simulink model "Modell_13_1_v2"  (R2018a)
settings: Solver=VariableStepAuto  StartTime=0.0  StopTime=10  MaxStep=0.001  RelTol=1e-3
libraries: simulink x2
settings Model: Creator=Uni  LastModifiedBy=Uni

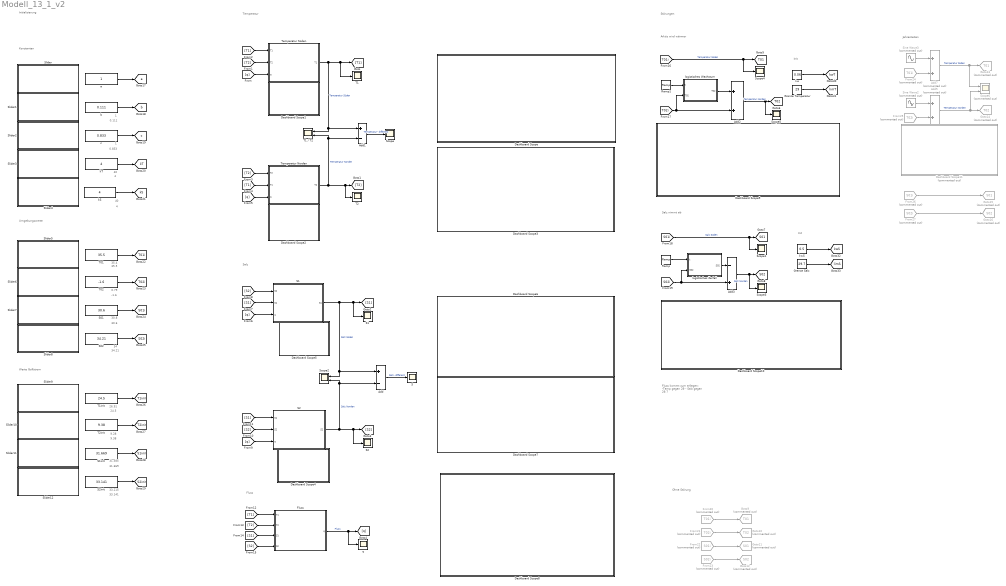
== system Modell_13_1_v2 ==
  note: 35.5
  note: -1.6
  note: 30.6
  note: 34.21
  note: 24.5
  note: 9.38
  note: 31.669
  note: 33.141
  note: 0.111
  note: 0.833
  note: 4
  note: 4
  note: Fluss kommt zum erliegen:
      | -Temp gegen 29
      | - Salz gegen 29.7
  note: Salz nimmt ab
  note: Ohne Störung
  note: Störungen
  note: 9.28
  note: 26.91
  note: 1
  note: 1
  note: 40
  note: 40
  note: 0.79
  note: 35.4
  note: 30.8
  note: 34
  note: 33.215
  note: 31.585
  note: Werte Golfstrom
  note: Umgebungswerte
  note: Konstanten
  note: Initialisierung
  note: Temperatur
  note: Salz
  note: Fluss
  note: Arktis wird wärmer
  note: Jahreszeiten
  note: Init
  note: Init
  Add : Sum  Inputs=+-
  Add1 : Sum  Inputs=+-
  Add2 : Sum
  Add3 : Sum  Inputs=-+
  Add5 : Sum  Commented=on
  Add7 : Sum  Commented=on
  Dashboard Scope : Subsystem  DialogController=hmiCreateDDGDialog  IsWebBlock=on  mask(MWDashboardBlock){webBlockId=232e5835-4ce7-4c9d-ab38-ef92145eaec7, webBlockType=sdiscope, ShowInitialText=on, HMISrcModelName=Modell_13_1_v2}
      mask prompts: webBlockId "WebBlock Id"; webBlockType "WebBlock Type"; HMISrcModelName "Source Model"
      mask help: SimulinkHMI:dialogs:HMIScopeDialogDesc
      mask Help: helpview([docroot '/mapfiles/simulink.map'], 'hmi_scope')
      mask Display:
      | if strcmp(get_param(bdroot(gcb),'BlockDiagramType'), 'library')
      |     image([(matlabroot) '/toolbox/simulink/hmi/icons/DashboardScope.png']);
      | end
  Dashboard Scope1 : Subsystem  DialogController=hmiCreateDDGDialog  IsWebBlock=on  mask(MWDashboardBlock){webBlockId=1d99596b-07c4-4ebe-b9bb-1a05cb83a3f7, webBlockType=sdiscope, ShowInitialText=on, HMISrcModelName=Modell_13_1_v2}
      mask prompts: webBlockId "WebBlock Id"; webBlockType "WebBlock Type"; HMISrcModelName "Source Model"
      mask help: SimulinkHMI:dialogs:HMIScopeDialogDesc
      mask Help: helpview([docroot '/mapfiles/simulink.map'], 'hmi_scope')
      mask Display:
      | if strcmp(get_param(bdroot(gcb),'BlockDiagramType'), 'library')
      |     image([(matlabroot) '/toolbox/simulink/hmi/icons/DashboardScope.png']);
      | end
  Dashboard Scope10 : Subsystem  DialogController=hmiCreateDDGDialog  IsWebBlock=on  mask(MWDashboardBlock){webBlockId=64694f84-10dd-4eec-98f6-5c1effd92336, webBlockType=sdiscope, ShowInitialText=on, HMISrcModelName=Modell_13_1_v2}
      mask prompts: webBlockId "WebBlock Id"; webBlockType "WebBlock Type"; HMISrcModelName "Source Model"
      mask help: SimulinkHMI:dialogs:HMIScopeDialogDesc
      mask Help: helpview([docroot '/mapfiles/simulink.map'], 'hmi_scope')
      mask Display:
      | if strcmp(get_param(bdroot(gcb),'BlockDiagramType'), 'library')
      |     image([(matlabroot) '/toolbox/simulink/hmi/icons/DashboardScope.png']);
      | end
  Dashboard Scope11 : Subsystem  Commented=on  DialogController=hmiCreateDDGDialog  IsWebBlock=on  mask(MWDashboardBlock){webBlockId=8f16ae8c-e240-448b-b23d-6ee9f960f799, webBlockType=sdiscope, ShowInitialText=on, HMISrcModelName=Modell_13_1_v2}
      mask prompts: webBlockId "WebBlock Id"; webBlockType "WebBlock Type"; HMISrcModelName "Source Model"
      mask help: SimulinkHMI:dialogs:HMIScopeDialogDesc
      mask Help: helpview([docroot '/mapfiles/simulink.map'], 'hmi_scope')
      mask Display:
      | if strcmp(get_param(bdroot(gcb),'BlockDiagramType'), 'library')
      |     image([(matlabroot) '/toolbox/simulink/hmi/icons/DashboardScope.png']);
      | end
  Dashboard Scope2 : Subsystem  DialogController=hmiCreateDDGDialog  IsWebBlock=on  mask(MWDashboardBlock){webBlockId=05d24440-a4cf-4944-9325-0dab2a17896c, webBlockType=sdiscope, ShowInitialText=on, HMISrcModelName=Modell_13_1_v2}
      mask prompts: webBlockId "WebBlock Id"; webBlockType "WebBlock Type"; HMISrcModelName "Source Model"
      mask help: SimulinkHMI:dialogs:HMIScopeDialogDesc
      mask Help: helpview([docroot '/mapfiles/simulink.map'], 'hmi_scope')
      mask Display:
      | if strcmp(get_param(bdroot(gcb),'BlockDiagramType'), 'library')
      |     image([(matlabroot) '/toolbox/simulink/hmi/icons/DashboardScope.png']);
      | end
  Dashboard Scope3 : Subsystem  DialogController=hmiCreateDDGDialog  IsWebBlock=on  mask(MWDashboardBlock){webBlockId=04dad841-fe90-4eb8-a8ca-631065159b5d, webBlockType=sdiscope, ShowInitialText=on, HMISrcModelName=Modell_13_1_v2}
      mask prompts: webBlockId "WebBlock Id"; webBlockType "WebBlock Type"; HMISrcModelName "Source Model"
      mask help: SimulinkHMI:dialogs:HMIScopeDialogDesc
      mask Help: helpview([docroot '/mapfiles/simulink.map'], 'hmi_scope')
      mask Display:
      | if strcmp(get_param(bdroot(gcb),'BlockDiagramType'), 'library')
      |     image([(matlabroot) '/toolbox/simulink/hmi/icons/DashboardScope.png']);
      | end
  Dashboard Scope4 : Subsystem  DialogController=hmiCreateDDGDialog  IsWebBlock=on  mask(MWDashboardBlock){webBlockId=a0aec621-b806-4cfe-bd24-7de60c6e42de, webBlockType=sdiscope, ShowInitialText=on, HMISrcModelName=Modell_13_1_v2}
      mask prompts: webBlockId "WebBlock Id"; webBlockType "WebBlock Type"; HMISrcModelName "Source Model"
      mask help: SimulinkHMI:dialogs:HMIScopeDialogDesc
      mask Help: helpview([docroot '/mapfiles/simulink.map'], 'hmi_scope')
      mask Display:
      | if strcmp(get_param(bdroot(gcb),'BlockDiagramType'), 'library')
      |     image([(matlabroot) '/toolbox/simulink/hmi/icons/DashboardScope.png']);
      | end
  Dashboard Scope5 : Subsystem  DialogController=hmiCreateDDGDialog  IsWebBlock=on  mask(MWDashboardBlock){webBlockId=6d85c72c-f90e-42d8-b24c-c4f45982be98, webBlockType=sdiscope, ShowInitialText=on, HMISrcModelName=Modell_13_1_v2}
      mask prompts: webBlockId "WebBlock Id"; webBlockType "WebBlock Type"; HMISrcModelName "Source Model"
      mask help: SimulinkHMI:dialogs:HMIScopeDialogDesc
      mask Help: helpview([docroot '/mapfiles/simulink.map'], 'hmi_scope')
      mask Display:
      | if strcmp(get_param(bdroot(gcb),'BlockDiagramType'), 'library')
      |     image([(matlabroot) '/toolbox/simulink/hmi/icons/DashboardScope.png']);
      | end
  Dashboard Scope6 : Subsystem  DialogController=hmiCreateDDGDialog  IsWebBlock=on  mask(MWDashboardBlock){webBlockId=292733d4-552e-447d-9455-c06405389df3, webBlockType=sdiscope, ShowInitialText=on, HMISrcModelName=Modell_13_1_v2}
      mask prompts: webBlockId "WebBlock Id"; webBlockType "WebBlock Type"; HMISrcModelName "Source Model"
      mask help: SimulinkHMI:dialogs:HMIScopeDialogDesc
      mask Help: helpview([docroot '/mapfiles/simulink.map'], 'hmi_scope')
      mask Display:
      | if strcmp(get_param(bdroot(gcb),'BlockDiagramType'), 'library')
      |     image([(matlabroot) '/toolbox/simulink/hmi/icons/DashboardScope.png']);
      | end
  Dashboard Scope7 : Subsystem  DialogController=hmiCreateDDGDialog  IsWebBlock=on  mask(MWDashboardBlock){webBlockId=c639261b-4e04-4c63-9ed6-005007be5a23, webBlockType=sdiscope, ShowInitialText=on, HMISrcModelName=Modell_13_1_v2}
      mask prompts: webBlockId "WebBlock Id"; webBlockType "WebBlock Type"; HMISrcModelName "Source Model"
      mask help: SimulinkHMI:dialogs:HMIScopeDialogDesc
      mask Help: helpview([docroot '/mapfiles/simulink.map'], 'hmi_scope')
      mask Display:
      | if strcmp(get_param(bdroot(gcb),'BlockDiagramType'), 'library')
      |     image([(matlabroot) '/toolbox/simulink/hmi/icons/DashboardScope.png']);
      | end
  Dashboard Scope8 : Subsystem  DialogController=hmiCreateDDGDialog  IsWebBlock=on  mask(MWDashboardBlock){webBlockId=c86a59e9-0323-4028-b559-a63c4fd5a7a8, webBlockType=sdiscope, ShowInitialText=on, HMISrcModelName=Modell_13_1_v2}
      mask prompts: webBlockId "WebBlock Id"; webBlockType "WebBlock Type"; HMISrcModelName "Source Model"
      mask help: SimulinkHMI:dialogs:HMIScopeDialogDesc
      mask Help: helpview([docroot '/mapfiles/simulink.map'], 'hmi_scope')
      mask Display:
      | if strcmp(get_param(bdroot(gcb),'BlockDiagramType'), 'library')
      |     image([(matlabroot) '/toolbox/simulink/hmi/icons/DashboardScope.png']);
      | end
  Dashboard Scope9 : Subsystem  DialogController=hmiCreateDDGDialog  IsWebBlock=on  mask(MWDashboardBlock){webBlockId=cec128b0-d988-4c21-801e-49592d9ce868, webBlockType=sdiscope, ShowInitialText=on, HMISrcModelName=Modell_13_1_v2}
      mask prompts: webBlockId "WebBlock Id"; webBlockType "WebBlock Type"; HMISrcModelName "Source Model"
      mask help: SimulinkHMI:dialogs:HMIScopeDialogDesc
      mask Help: helpview([docroot '/mapfiles/simulink.map'], 'hmi_scope')
      mask Display:
      | if strcmp(get_param(bdroot(gcb),'BlockDiagramType'), 'library')
      |     image([(matlabroot) '/toolbox/simulink/hmi/icons/DashboardScope.png']);
      | end
  Fluss : Subsystem
  From20 : From  Commented=on  GotoTag=T01i  TagVisibility=global
  From21 : From  Commented=on  GotoTag=T02i  TagVisibility=global
  From22 : From  Commented=on  GotoTag=S01i  TagVisibility=global
  From23 : From  Commented=on  GotoTag=S02i  TagVisibility=global
  From24 : From  Commented=on  GotoTag=T01i  TagVisibility=global
  From25 : From  Commented=on  GotoTag=T02i  TagVisibility=global
  From26 : From  Commented=on  GotoTag=S01i  TagVisibility=global
  From27 : From  Commented=on  GotoTag=S02i  TagVisibility=global
  Goto10 : Goto  Commented=on  GotoTag=T02  TagVisibility=global
  Goto11 : Goto  Commented=on  GotoTag=S01  TagVisibility=global
  Goto12 : Goto  Commented=on  GotoTag=S02  TagVisibility=global
  Goto13 : Goto  Commented=on  GotoTag=T01  TagVisibility=global
  Goto14 : Goto  Commented=on  GotoTag=T02  TagVisibility=global
  Goto15 : Goto  Commented=on  GotoTag=S01  TagVisibility=global
  Goto16 : Goto  Commented=on  GotoTag=S02  TagVisibility=global
  Goto9 : Goto  Commented=on  GotoTag=T01  TagVisibility=global
  Grenze Temperatur : Constant  Value=29
  Grenze Salz : Constant  Value=29.7
  Ramp : simulink/Sources/Ramp  slope=1  start=0  InitialOutput=0
  Ramp1 : simulink/Sources/Ramp  slope=1  start=0  InitialOutput=0
  S : Scope
  S01 : Constant  Value=30.6
  S02 : Constant  Value=34.21
  S1 : Scope
  "S1 " : Subsystem
  S1init : Constant  Value=31.669
  S2 : Scope
  "S2 " : Subsystem
  S2init : Constant  Value=33.141
  Scope{,1,3..5} (5 alike) : Scope
  Scope2 : Scope  NumInputPorts=2
  Scope6 : Scope  Commented=on  NumInputPorts=2
  Sine Wave2 : Sin  Commented=on  Amplitude=0.5  Bias=+3  Frequency=2*pi  Phase=-pi/2  SampleTime=0
  Sine Wave3 : Sin  Commented=on  Amplitude=4.5  Bias=-10  Frequency=2*pi  Phase=-pi/2  SampleTime=0
  Slider : Subsystem  DialogController=hmiCreateDDGDialog  IsWebBlock=on  mask(MWDashboardBlock){webBlockId=1194ebb6-db82-4b45-8843-debe8bbaaa56, webBlockType=slider, ShowInLibBrowser=on, ShowInitialText=on, HMISrcModelName=Modell_13_1_v2}
      mask prompts: webBlockId "WebBlock Id"; webBlockType "WebBlock Type"; HMISrcModelName "Source Model"
      mask help: SimulinkHMI:dialogs:SliderDialogDesc
      mask Help: helpview([docroot '/mapfiles/simulink.map'], 'hmi_slider')
      mask Display:
      | if strcmp(get_param(bdroot(gcb),'BlockDiagramType'), 'library')
      |     image([(matlabroot) '/toolbox/simulink/hmi/icons/Slider.png']);
      | end
  Slider1 : Subsystem  DialogController=hmiCreateDDGDialog  IsWebBlock=on  mask(MWDashboardBlock){webBlockId=a4277e18-3754-400d-9202-f3c74c830cee, webBlockType=slider, ShowInLibBrowser=on, ShowInitialText=on, HMISrcModelName=Modell_13_1_v2}
      mask prompts: webBlockId "WebBlock Id"; webBlockType "WebBlock Type"; HMISrcModelName "Source Model"
      mask help: SimulinkHMI:dialogs:SliderDialogDesc
      mask Help: helpview([docroot '/mapfiles/simulink.map'], 'hmi_slider')
      mask Display:
      | if strcmp(get_param(bdroot(gcb),'BlockDiagramType'), 'library')
      |     image([(matlabroot) '/toolbox/simulink/hmi/icons/Slider.png']);
      | end
  Slider10 : Subsystem  DialogController=hmiCreateDDGDialog  IsWebBlock=on  mask(MWDashboardBlock){webBlockId=a224fc53-c758-4af3-a825-d89d70dab4de, webBlockType=slider, ShowInLibBrowser=on, ShowInitialText=on, HMISrcModelName=Modell_13_1_v2}
      mask prompts: webBlockId "WebBlock Id"; webBlockType "WebBlock Type"; HMISrcModelName "Source Model"
      mask help: SimulinkHMI:dialogs:SliderDialogDesc
      mask Help: helpview([docroot '/mapfiles/simulink.map'], 'hmi_slider')
      mask Display:
      | if strcmp(get_param(bdroot(gcb),'BlockDiagramType'), 'library')
      |     image([(matlabroot) '/toolbox/simulink/hmi/icons/Slider.png']);
      | end
  Slider11 : Subsystem  DialogController=hmiCreateDDGDialog  IsWebBlock=on  mask(MWDashboardBlock){webBlockId=208660da-0c53-427b-b493-98923b800816, webBlockType=slider, ShowInLibBrowser=on, ShowInitialText=on, HMISrcModelName=Modell_13_1_v2}
      mask prompts: webBlockId "WebBlock Id"; webBlockType "WebBlock Type"; HMISrcModelName "Source Model"
      mask help: SimulinkHMI:dialogs:SliderDialogDesc
      mask Help: helpview([docroot '/mapfiles/simulink.map'], 'hmi_slider')
      mask Display:
      | if strcmp(get_param(bdroot(gcb),'BlockDiagramType'), 'library')
      |     image([(matlabroot) '/toolbox/simulink/hmi/icons/Slider.png']);
      | end
  Slider12 : Subsystem  DialogController=hmiCreateDDGDialog  IsWebBlock=on  mask(MWDashboardBlock){webBlockId=a21bbc8b-4054-4a71-80f2-ee0f79f54661, webBlockType=slider, ShowInLibBrowser=on, ShowInitialText=on, HMISrcModelName=Modell_13_1_v2}
      mask prompts: webBlockId "WebBlock Id"; webBlockType "WebBlock Type"; HMISrcModelName "Source Model"
      mask help: SimulinkHMI:dialogs:SliderDialogDesc
      mask Help: helpview([docroot '/mapfiles/simulink.map'], 'hmi_slider')
      mask Display:
      | if strcmp(get_param(bdroot(gcb),'BlockDiagramType'), 'library')
      |     image([(matlabroot) '/toolbox/simulink/hmi/icons/Slider.png']);
      | end
  Slider2 : Subsystem  DialogController=hmiCreateDDGDialog  IsWebBlock=on  mask(MWDashboardBlock){webBlockId=08e3c6e8-cebd-46e9-85f5-789084b6eeee, webBlockType=slider, ShowInLibBrowser=on, ShowInitialText=on, HMISrcModelName=Modell_13_1_v2}
      mask prompts: webBlockId "WebBlock Id"; webBlockType "WebBlock Type"; HMISrcModelName "Source Model"
      mask help: SimulinkHMI:dialogs:SliderDialogDesc
      mask Help: helpview([docroot '/mapfiles/simulink.map'], 'hmi_slider')
      mask Display:
      | if strcmp(get_param(bdroot(gcb),'BlockDiagramType'), 'library')
      |     image([(matlabroot) '/toolbox/simulink/hmi/icons/Slider.png']);
      | end
  Slider3 : Subsystem  DialogController=hmiCreateDDGDialog  IsWebBlock=on  mask(MWDashboardBlock){webBlockId=50bb7ae8-36da-4efa-9e34-4aa5702c7458, webBlockType=slider, ShowInLibBrowser=on, ShowInitialText=on, HMISrcModelName=Modell_13_1_v2}
      mask prompts: webBlockId "WebBlock Id"; webBlockType "WebBlock Type"; HMISrcModelName "Source Model"
      mask help: SimulinkHMI:dialogs:SliderDialogDesc
      mask Help: helpview([docroot '/mapfiles/simulink.map'], 'hmi_slider')
      mask Display:
      | if strcmp(get_param(bdroot(gcb),'BlockDiagramType'), 'library')
      |     image([(matlabroot) '/toolbox/simulink/hmi/icons/Slider.png']);
      | end
  Slider4 : Subsystem  DialogController=hmiCreateDDGDialog  IsWebBlock=on  mask(MWDashboardBlock){webBlockId=76cd73b1-19c3-4efe-a0c8-12da85b53291, webBlockType=slider, ShowInLibBrowser=on, ShowInitialText=on, HMISrcModelName=Modell_13_1_v2}
      mask prompts: webBlockId "WebBlock Id"; webBlockType "WebBlock Type"; HMISrcModelName "Source Model"
      mask help: SimulinkHMI:dialogs:SliderDialogDesc
      mask Help: helpview([docroot '/mapfiles/simulink.map'], 'hmi_slider')
      mask Display:
      | if strcmp(get_param(bdroot(gcb),'BlockDiagramType'), 'library')
      |     image([(matlabroot) '/toolbox/simulink/hmi/icons/Slider.png']);
      | end
  Slider5 : Subsystem  DialogController=hmiCreateDDGDialog  IsWebBlock=on  mask(MWDashboardBlock){webBlockId=7cffd9e6-a6a1-4812-b39f-a26ba2170319, webBlockType=slider, ShowInLibBrowser=on, ShowInitialText=on, HMISrcModelName=Modell_13_1_v2}
      mask prompts: webBlockId "WebBlock Id"; webBlockType "WebBlock Type"; HMISrcModelName "Source Model"
      mask help: SimulinkHMI:dialogs:SliderDialogDesc
      mask Help: helpview([docroot '/mapfiles/simulink.map'], 'hmi_slider')
      mask Display:
      | if strcmp(get_param(bdroot(gcb),'BlockDiagramType'), 'library')
      |     image([(matlabroot) '/toolbox/simulink/hmi/icons/Slider.png']);
      | end
  Slider6 : Subsystem  DialogController=hmiCreateDDGDialog  IsWebBlock=on  mask(MWDashboardBlock){webBlockId=ae5c7515-8043-4fa6-9881-f68136f0045e, webBlockType=slider, ShowInLibBrowser=on, ShowInitialText=on, HMISrcModelName=Modell_13_1_v2}
      mask prompts: webBlockId "WebBlock Id"; webBlockType "WebBlock Type"; HMISrcModelName "Source Model"
      mask help: SimulinkHMI:dialogs:SliderDialogDesc
      mask Help: helpview([docroot '/mapfiles/simulink.map'], 'hmi_slider')
      mask Display:
      | if strcmp(get_param(bdroot(gcb),'BlockDiagramType'), 'library')
      |     image([(matlabroot) '/toolbox/simulink/hmi/icons/Slider.png']);
      | end
  Slider7 : Subsystem  DialogController=hmiCreateDDGDialog  IsWebBlock=on  mask(MWDashboardBlock){webBlockId=fc529bb9-da36-454c-b7af-e469445be323, webBlockType=slider, ShowInLibBrowser=on, ShowInitialText=on, HMISrcModelName=Modell_13_1_v2}
      mask prompts: webBlockId "WebBlock Id"; webBlockType "WebBlock Type"; HMISrcModelName "Source Model"
      mask help: SimulinkHMI:dialogs:SliderDialogDesc
      mask Help: helpview([docroot '/mapfiles/simulink.map'], 'hmi_slider')
      mask Display:
      | if strcmp(get_param(bdroot(gcb),'BlockDiagramType'), 'library')
      |     image([(matlabroot) '/toolbox/simulink/hmi/icons/Slider.png']);
      | end
  Slider8 : Subsystem  DialogController=hmiCreateDDGDialog  IsWebBlock=on  mask(MWDashboardBlock){webBlockId=21e985ee-664e-47b4-a928-9d2b18b75e43, webBlockType=slider, ShowInLibBrowser=on, ShowInitialText=on, HMISrcModelName=Modell_13_1_v2}
      mask prompts: webBlockId "WebBlock Id"; webBlockType "WebBlock Type"; HMISrcModelName "Source Model"
      mask help: SimulinkHMI:dialogs:SliderDialogDesc
      mask Help: helpview([docroot '/mapfiles/simulink.map'], 'hmi_slider')
      mask Display:
      | if strcmp(get_param(bdroot(gcb),'BlockDiagramType'), 'library')
      |     image([(matlabroot) '/toolbox/simulink/hmi/icons/Slider.png']);
      | end
  Slider9 : Subsystem  DialogController=hmiCreateDDGDialog  IsWebBlock=on  mask(MWDashboardBlock){webBlockId=ac2e80ed-5c91-407a-8dd2-6c7a8cc22064, webBlockType=slider, ShowInLibBrowser=on, ShowInitialText=on, HMISrcModelName=Modell_13_1_v2}
      mask prompts: webBlockId "WebBlock Id"; webBlockType "WebBlock Type"; HMISrcModelName "Source Model"
      mask help: SimulinkHMI:dialogs:SliderDialogDesc
      mask Help: helpview([docroot '/mapfiles/simulink.map'], 'hmi_slider')
      mask Display:
      | if strcmp(get_param(bdroot(gcb),'BlockDiagramType'), 'library')
      |     image([(matlabroot) '/toolbox/simulink/hmi/icons/Slider.png']);
      | end
  T01 : Constant  Value=35.5
  T02 : Constant  Value=-1.6
  T1 : Scope
  T1 / T2 : Scope  NumInputPorts=2
  T1init : Constant  Value=24.5
  "T2 " : Scope
  T2init : Constant  Value=9.38
  Temperatur Norden : Subsystem
  Temperatur Süden : Subsystem
  a : Constant
  b : Constant  Value=0.111
  c : Constant  Value=0.833
  kS : Constant  Value=4
  kT : Constant  Value=4
  kw : Constant  Value=0.06
  kwS : Constant  Value=0.5
  logistisches Wachstum : Subsystem
  logistisches Zerfall : Subsystem
  q : Scope
  tag scope: S01=global, S01i=global, S02=global, S02i=global, S1init=global, S2init=global, T01=global, T01i=global, T02=global, T02i=global, T1init=global, T2init=global, a=global, b=global, c=global, kS=global, kT=global, kwS=global, kwT=global, limS=global, limT=global
  wires:
  [T1] -> Temperatur Süden/1("T1 ")
  [T2] -> Temperatur Süden/2("T2 ")
  [q] -> Temperatur Süden/3("q ")
  Temperatur Süden/1(T1) -> T1/1, [T1], T1 / T2/1, Add1/1  "Temperatur Süden"
  Temperatur Norden/1("T2 ") -> T1 / T2/2, Add1/2, "T2 "/1, [T2]  "Temperatur Norden"
  [T2] -> Temperatur Norden/1("T2  ")
  [T1] -> Temperatur Norden/2(T1)
  [q] -> Temperatur Norden/3("q ")
  [S2] -> "S1 "/1(S2)
  [S1] -> "S1 "/2("S1 ")
  [q] -> "S1 "/3(q)
  "S1 "/1(S1) -> S1/1, [S1], Add/1, Scope2/1  "Salz Süden"
  [q] -> "S2 "/3(q)
  "S2 "/1(S2) -> S2/1, [S2], Add/2, Scope2/2  "Salz Norden"
  [S2] -> "S2 "/2("S2 ")
  [S1] -> "S2 "/1("S1 ")
  [T1] -> Fluss/1(T1)
  [T2] -> Fluss/2(T2)
  [S1] -> Fluss/3(S1)
  [S2] -> Fluss/4(S2)
  Add1/1 -> Scope/1  "Temperatur- differenz"
  [S01i] -> Scope1/1, [S01]  "Salz Süden"
  Add3/1 -> Scope3/1, [S02]  "Salz Norden"
  Add7/1 -> Scope6/1, Goto13/1  "Temperatur Süden"
  From24/1 -> Add7/2
  From25/1 -> Add5/2
  From26/1 -> Goto15/1
  Add5/1 -> Scope6/2, Goto14/1  "Temperatur Norden"
  Sine Wave3/1 -> Add7/1
  Sine Wave2/1 -> Add5/1
  From27/1 -> Goto16/1
  [T01i] -> Scope4/1, [T01]  "Temperatur Süden"
  Ramp1/1 -> logistisches Wachstum/1(t)
  [T02i] -> logistisches Wachstum/2("T02 "), Add2/2
  logistisches Wachstum/1(T02) -> Add2/1
  Add2/1 -> Scope5/1, [T02]  "Temperatur Norden"
  logistisches Zerfall/1(S02) -> Add3/1
  [S02i] -> Add3/2, logistisches Zerfall/2("S02 ")
  Ramp/1 -> logistisches Zerfall/1(t)
  Fluss/1(q) -> q/1, [q]  "Fluss"
  a/1 -> [a]
  b/1 -> [b]
  c/1 -> [c]
  kT/1 -> [kT]
  kS/1 -> [kS]
  T01/1 -> [T01i]
  T02/1 -> [T02i]
  S01/1 -> [S01i]
  S02/1 -> [S02i]
  S2init/1 -> [S2init]
  S1init/1 -> [S1init]
  T2init/1 -> [T2init]
  T1init/1 -> [T1init]
  From20/1 -> Goto9/1
  From21/1 -> Goto10/1
  From22/1 -> Goto11/1
  From23/1 -> Goto12/1
  Grenze Temperatur/1 -> [limT]
  kw/1 -> [kwT]
  Grenze Salz/1 -> [limS]
  kwS/1 -> [kwS]
  Add/1 -> S/1  "Salz- differenz"

== system Modell_13_1_v2/Dashboard Scope ==

== system Modell_13_1_v2/Dashboard Scope1 ==

== system Modell_13_1_v2/Dashboard Scope10 ==

== system Modell_13_1_v2/Dashboard Scope11 ==

== system Modell_13_1_v2/Dashboard Scope2 ==

== system Modell_13_1_v2/Dashboard Scope3 ==

== system Modell_13_1_v2/Dashboard Scope4 ==

== system Modell_13_1_v2/Dashboard Scope5 ==

== system Modell_13_1_v2/Dashboard Scope6 ==

== system Modell_13_1_v2/Dashboard Scope7 ==

== system Modell_13_1_v2/Dashboard Scope8 ==

== system Modell_13_1_v2/Dashboard Scope9 ==

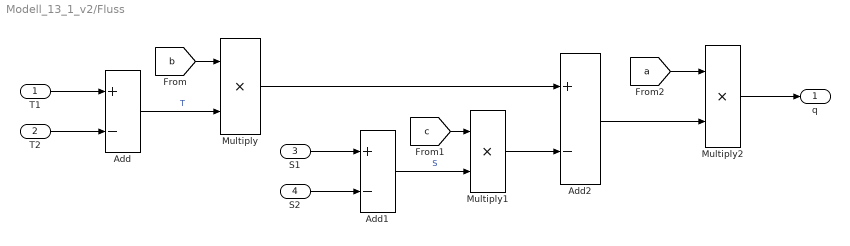
== system Modell_13_1_v2/Fluss ==
  T1 : Inport
  T2 : Inport  Port=2
  S1 : Inport  Port=3
  S2 : Inport  Port=4
  Add : Sum  Inputs=+-
  Add1 : Sum  Inputs=+-
  Add2 : Sum  Inputs=+-
  Multiply : Product
  Multiply1 : Product
  Multiply2 : Product
  q : Outport
  wires:
  Add/1 -> Multiply/2  "T"
  [a] -> Multiply2/1
  Add1/1 -> Multiply1/2  "S"
  [c] -> Multiply1/1
  Multiply2/1 -> q/1
  Multiply/1 -> Add2/1
  Add2/1 -> Multiply2/2
  Multiply1/1 -> Add2/2
  [b] -> Multiply/1
  T1/1 -> Add/1
  T2/1 -> Add/2
  S2/1 -> Add1/2
  S1/1 -> Add1/1

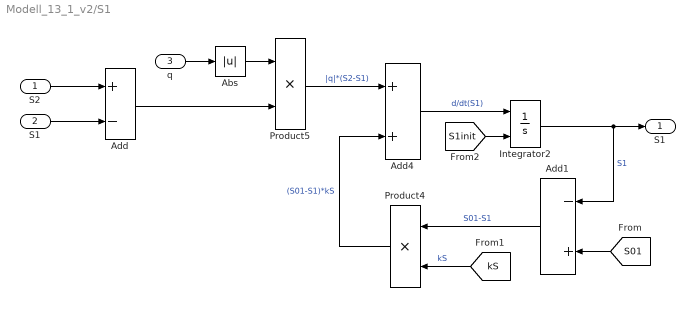
== system Modell_13_1_v2/S1  ==
  S2 : Inport
  "S1 " : Inport  Port=2
  q : Inport  Port=3
  Abs : Abs
  Add : Sum  Inputs=+-
  Add1 : Sum  Inputs=-+
  Add4 : Sum
  Integrator2 : Integrator  InitialConditionSource=external
  Product4 : Product
  Product5 : Product
  S1 : Outport
  wires:
  q/1 -> Abs/1
  Product4/1 -> Add4/2  "(S01-S1)*kS"
  Integrator2/1 -> S1/1, Add1/1  "S1"
  Add4/1 -> Integrator2/1  "d/dt(S1)"
  Product5/1 -> Add4/1  "|q|*(S2-S1)"
  Add/1 -> Product5/2
  Add1/1 -> Product4/1  "S01-S1"
  [S01] -> Add1/2
  S2/1 -> Add/1
  [S1init] -> Integrator2/2
  [kS] -> Product4/2  "kS"
  "S1 "/1 -> Add/2
  Abs/1 -> Product5/1

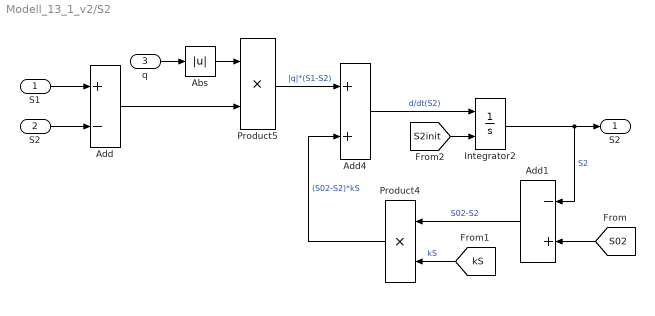
== system Modell_13_1_v2/S2  ==
  "S1 " : Inport
  "S2 " : Inport  Port=2
  q : Inport  Port=3
  Abs : Abs
  Add : Sum  Inputs=+-
  Add1 : Sum  Inputs=-+
  Add4 : Sum
  Integrator2 : Integrator  InitialConditionSource=external
  Product4 : Product
  Product5 : Product
  S2 : Outport
  wires:
  q/1 -> Abs/1
  Product4/1 -> Add4/2  "(S02-S2)*kS"
  Integrator2/1 -> S2/1, Add1/1  "S2"
  Add4/1 -> Integrator2/1  "d/dt(S2)"
  Product5/1 -> Add4/1  "|q|*(S1-S2)"
  Add/1 -> Product5/2
  Add1/1 -> Product4/1  "S02-S2"
  "S1 "/1 -> Add/1
  [S2init] -> Integrator2/2
  [kS] -> Product4/2  "kS"
  "S2 "/1 -> Add/2
  Abs/1 -> Product5/1
  [S02] -> Add1/2

== system Modell_13_1_v2/Slider ==

== system Modell_13_1_v2/Slider1 ==

== system Modell_13_1_v2/Slider10 ==

== system Modell_13_1_v2/Slider11 ==

== system Modell_13_1_v2/Slider12 ==

== system Modell_13_1_v2/Slider2 ==

== system Modell_13_1_v2/Slider3 ==

== system Modell_13_1_v2/Slider4 ==

== system Modell_13_1_v2/Slider5 ==

== system Modell_13_1_v2/Slider6 ==

== system Modell_13_1_v2/Slider7 ==

== system Modell_13_1_v2/Slider8 ==

== system Modell_13_1_v2/Slider9 ==

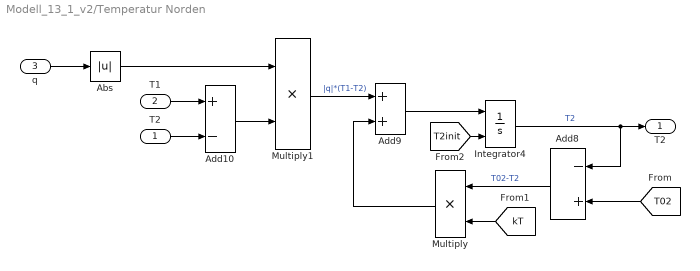
== system Modell_13_1_v2/Temperatur Norden ==
  "T2  " : Inport
  T1 : Inport  Port=2
  "q " : Inport  Port=3
  Abs : Abs
  Add10 : Sum  Inputs=+-
  Add8 : Sum  Inputs=-+
  Add9 : Sum
  Integrator4 : Integrator  InitialConditionSource=external
  Multiply : Product
  Multiply1 : Product
  "T2 " : Outport
  wires:
  Add8/1 -> Multiply/1  "T02-T2"
  Multiply1/1 -> Add9/1  "|q|*(T1-T2)"
  [kT] -> Multiply/2
  Add10/1 -> Multiply1/2
  "q "/1 -> Abs/1
  [T2init] -> Integrator4/2
  Multiply/1 -> Add9/2
  Integrator4/1 -> Add8/1, "T2 "/1  "T2"
  Add9/1 -> Integrator4/1
  [T02] -> Add8/2
  "T2  "/1 -> Add10/2
  T1/1 -> Add10/1
  Abs/1 -> Multiply1/1

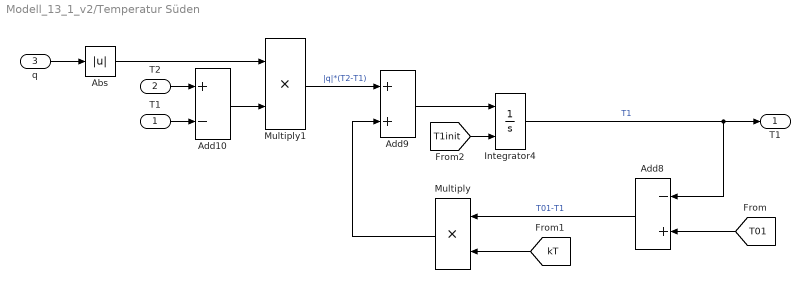
== system Modell_13_1_v2/Temperatur Süden ==
  "T1 " : Inport
  "T2 " : Inport  Port=2
  "q " : Inport  Port=3
  Abs : Abs
  Add10 : Sum  Inputs=+-
  Add8 : Sum  Inputs=-+
  Add9 : Sum
  Integrator4 : Integrator  InitialConditionSource=external
  Multiply : Product
  Multiply1 : Product
  T1 : Outport
  wires:
  Add8/1 -> Multiply/1  "T01-T1"
  Multiply1/1 -> Add9/1  "|q|*(T2-T1)"
  [kT] -> Multiply/2
  Add10/1 -> Multiply1/2
  "q "/1 -> Abs/1
  [T1init] -> Integrator4/2
  Multiply/1 -> Add9/2
  Integrator4/1 -> T1/1, Add8/1  "T1"
  Add9/1 -> Integrator4/1
  [T01] -> Add8/2
  "T1 "/1 -> Add10/2
  "T2 "/1 -> Add10/1
  Abs/1 -> Multiply1/1

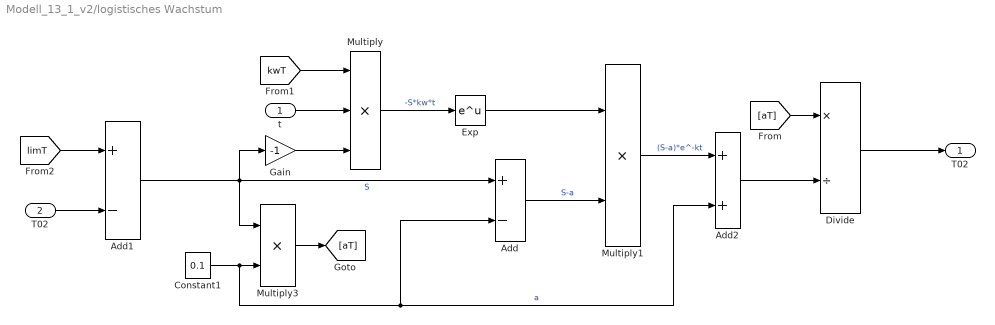
== system Modell_13_1_v2/logistisches Wachstum ==
  t : Inport
  "T02 " : Inport  Port=2
  Add : Sum  Inputs=+-
  Add1 : Sum  Inputs=+-
  Add2 : Sum
  Constant1 : Constant  Value=0.1
  Divide : Product  Inputs=*/
  Exp : Math  SaturateOnIntegerOverflow=on
  Gain : Gain  Gain=-1
  Multiply : Product  Inputs=3
  Multiply1 : Product
  Multiply3 : Product
  T02 : Outport
  wires:
  [kwT] -> Multiply/1
  t/1 -> Multiply/2
  Multiply/1 -> Exp/1  "-S*kw*t"
  Exp/1 -> Multiply1/1
  Multiply1/1 -> Add2/1  "(S-a)*e^-kt"
  Divide/1 -> T02/1
  Add/1 -> Multiply1/2  "S-a"
  Constant1/1 -> Add/2, Add2/2, Multiply3/2  "a"
  Add1/1 -> Add/1, Multiply3/1, Gain/1  "S"
  Gain/1 -> Multiply/3
  Multiply3/1 -> [aT]
  Add2/1 -> Divide/2
  [aT] -> Divide/1
  [limT] -> Add1/1
  "T02 "/1 -> Add1/2

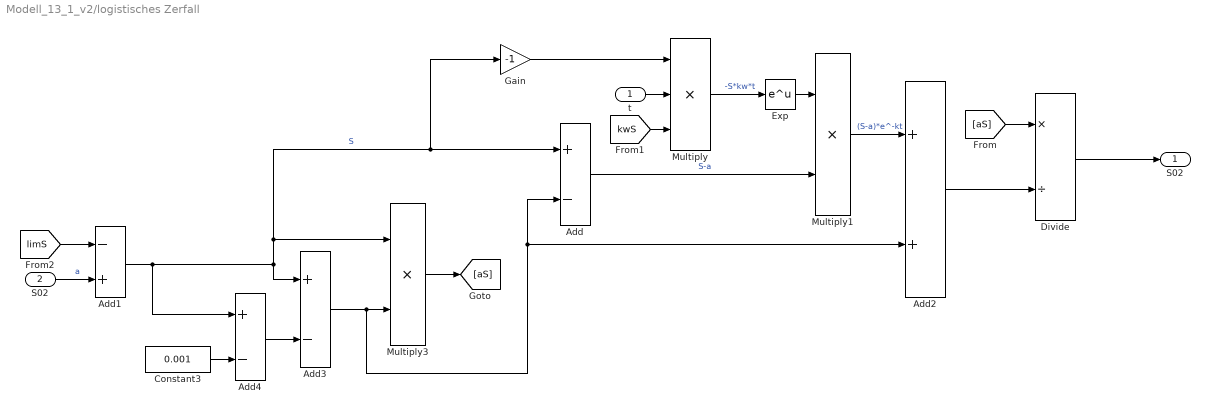
== system Modell_13_1_v2/logistisches Zerfall ==
  t : Inport
  "S02 " : Inport  Port=2
  Add : Sum  Inputs=+-
  Add1 : Sum  Inputs=-+
  Add2 : Sum
  Add3 : Sum  Inputs=+-
  Add4 : Sum  Inputs=+-
  Constant3 : Constant  Value=0.001
  Divide : Product  Inputs=*/
  Exp : Math  SaturateOnIntegerOverflow=on
  Gain : Gain  Gain=-1
  Multiply : Product  Inputs=3
  Multiply1 : Product
  Multiply3 : Product
  S02 : Outport
  wires:
  [kwS] -> Multiply/3
  t/1 -> Multiply/2
  Multiply/1 -> Exp/1  "-S*kw*t"
  Exp/1 -> Multiply1/1
  Multiply1/1 -> Add2/1  "(S-a)*e^-kt"
  Divide/1 -> S02/1
  Add/1 -> Multiply1/2  "S-a"
  "S02 "/1 -> Add1/2  "a"
  Add1/1 -> Add3/1, Gain/1, Add/1, Multiply3/1, Add4/1  "S"
  Multiply3/1 -> [aS]
  Add2/1 -> Divide/2
  [aS] -> Divide/1
  [limS] -> Add1/1
  Add3/1 -> Multiply3/2, Add2/2, Add/2
  Gain/1 -> Multiply/1
  Constant3/1 -> Add4/2
  Add4/1 -> Add3/2
